simulink model "purepursuit"  (R2025a)
settings: Solver=VariableStepAuto  StartTime=0.0  StopTime=200  RelTol=1e-3
libraries: drivingscenarioandsensors x1, autolibshared x1
settings Model: Creator=bsb  LastModifiedBy=bsb

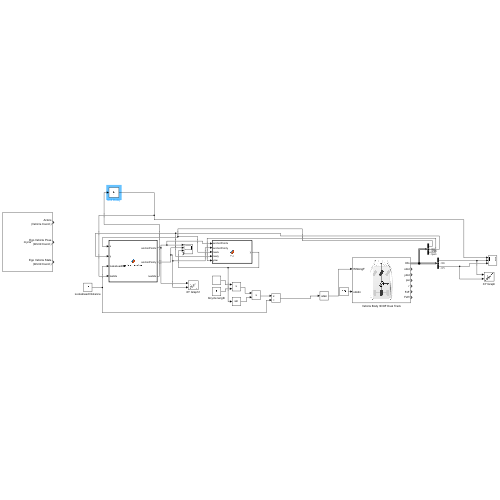
[thumbnail: Simulink's stored preview of the top-level diagram]
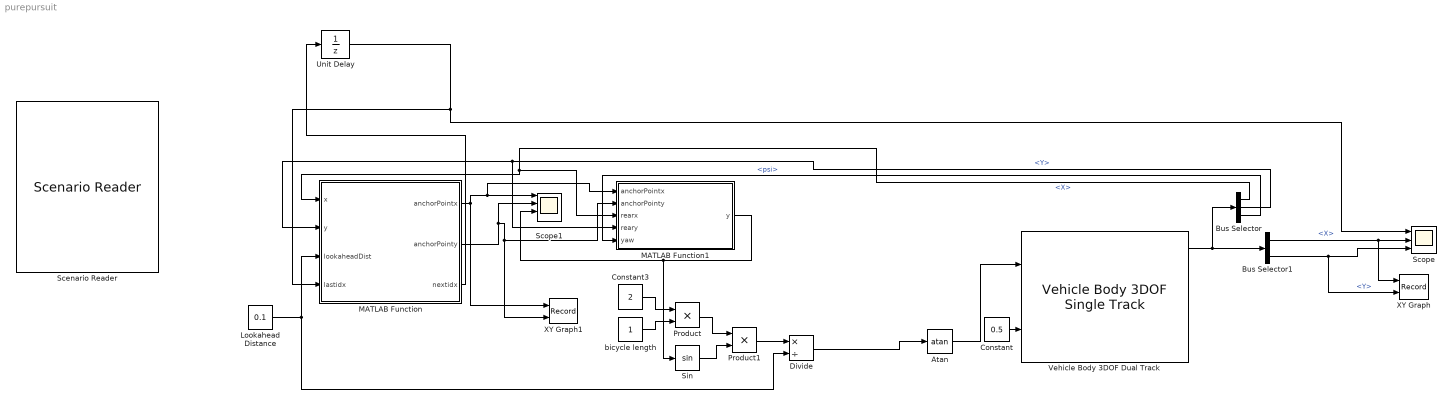
== system purepursuit ==
  Atan : Trigonometry  Operator=atan
  Bus Selector : BusSelector  OutputSignals=InertFrm.RearAxl.Disp.X,InertFrm.RearAxl.Disp.Y,InertFrm.Cg.Ang.psi
  Bus Selector1 : BusSelector  OutputSignals=InertFrm.Cg.Disp.X,InertFrm.Cg.Disp.Y
  Constant : Constant  Value=0.5
  Constant3 : Constant  Value=2
  Divide : Product  Inputs=*/
  Lookahead Distance : Constant  Value=0.1
  MATLAB Function : MATLAB Function  TreatAsAtomicUnit=on
  MATLAB Function1 : MATLAB Function  TreatAsAtomicUnit=on
  Product : Product
  Product1 : Product
  Scenario Reader : drivingscenarioandsensors/Scenario Reader  ScenarioSource=From file  ScenarioFileName=C:\Users\bsb\Documents\MATLAB\mycar.mat  ScenarioVariableName=scenario  OutputCoordinateSystem=Vehicle coordinates  EgoVehicleSource=Scenario  EgoVehicleActorID=1  OrientVehiclesOnRoad=off  OutputEgoVehiclePose=on  OutputEgoVehicleState=on  SampleTime=0.1  LaneBoundaryOutput=None  LaneBoundaryDistance=0:0.5:9.5  LaneBoundaryLocation=Center of lane markings  BusNameSource=Auto  BusName=BusActors  BusNumActorsSource=Scenario  BusNumActors=100  BusName2Source=Auto  BusName2=BusLaneBoundaries  BusNumLaneBoundariesSource=Scenario  BusNumLaneBoundaries=10  BusName3Source=Auto  BusName3=BusEgoActor  BusName4Source=Auto  BusName4=BusEgoState  ShowCoordinateLabels=on  SimulateUsing=Interpreted execution
  Scope : Scope  NumInputPorts=3
      settings: ActiveDisplayYMinimum=6.6611816133990995  ActiveDisplayYMaximum=22.945488903629986
  Scope1 : Scope  NumInputPorts=4
      settings: ActiveDisplayYMinimum=-0.018595181239648123  ActiveDisplayYMaximum=0.00095474296248539321
  Sin : Trigonometry
  Unit Delay : UnitDelay  SampleTime=-1  HasFrameUpgradeWarning=on
  Vehicle Body 3DOF Dual Track : autolibshared/Vehicle Body 3DOF Single Track  trackMode=Single (bicycle)  inputMode=External longitudinal velocity  frontSteerMode=on  rearSteerMode=off  windMode=off  muMode=off  extFMode=off  extMMode=off  htchFMode=off  htchMMode=off  extXo=off  extpsio=off  extxdoto=off  extro=off  extYo=off  extTamb=off  extydoto=off  aMode=2  NF=2  NR=2  m=2000  a=1.4  b=1.6  h=0.35  dh=1  hh=0.2  X_o=0  xdot_o=0  CalphaMode=off  sigmaMode=on  d=0  hl=0  w=[1.4,1.4]  Cy_f=12e3  Cy_r=11e3  sigma_f=.1  sigma_r=.1  alpha_f_brk=[-.1 .1]  Cy_f_data=[-9e3 9e3]  alpha_r_brk=[-.1 .1]  Cy_r_data=[-9e3 9e3]  Y_o=0  ydot_o=0  Izz=4000  psi_o=0  r_o=0  Af=2  Cd=.3  Cl=.1  Cpm=.1  beta_w=[0 0.01:0.01:0.3]  Cs=[0:0.03:0.9]  Cym=[0 1e-6:0.01:0.3]  Pabs=101325  Tair=273  g=9.81  mu=1  xdot_tol=.01  Fznom=5000  Fxtire_sat=7e4  Fytire_sat=7e4  longOff=0  latOff=0  vertOff=0  wrapAng=off
      settings: LibrarySourceBlock=vehdynlibeom/Vehicle Body 3DOF Dual Track
  XY Graph : Record  NumPorts=2.0  FileSettingsInternal="{\"entries\":[{\"content\":{\"excelSettings\":{\"content\":{},\"type\":\"Streamout.ExcelSettings\"},\"parquetSettings\":{\"content\":{},\"type\":\"Streamout.ParquetSettings\"}},\"type\":\"Streamout.FileSettingStorage\",\"uuid\":\"\"}],\"packageUris\":[\"http:\\/\\/schema.mathworks.com\\/mf0\\/streamout_blocks\\/R2020a\"],\"version\":\"1.0\"}"  FrameSettings=[0, 0]  Layout=[1 1]  SignalsInternal="{\"entries\":[{\"content\":{\"signals\":[{\"content\":{\"blockPath\":[],\"dimensions\":[1],\"domain\":\"\",\"lineColor\":\"#a2142f\",\"plots\":[ 1 ],\"port\":1,\"sid\":[\"\"],\"signalID\":1,\"signalName\":\"<X>\"},\"type\":\"RecordBlkView.Signal\",\"uuid\":\"\"},{\"content\":{\"blockPath\":[],\"dimensions\":[1],\"domain\":\"\",\"lineColor\":\"#139fff\",\"plots\":[ 1 ],\"port\":2,\"sid\":[\"\"],\"signalID\":2,\"signalName\":\"<Y>\"},\"type\":\"RecordBlkView.Signal\",\"uuid\":\"\"}]},\"type\":\"RecordBlkView.InputSignals\",\"uuid\":\"\"}],\"packageUris\":[\"http:\\/\\/schema.mathworks.com\\/mf0\\/streamout_blocks\\/R2020a\"],\"version\":\"1.0\"}"  VisualizationBindings="{\"xyplotplugin\":{\"info\":[{\"series\":[{\"bindingParametersList\":[{\"parameter\":\"X-Axis\",\"signalID\":1,\"signalName\":\"<X>\"},{\"parameter\":\"Y-Axis\",\"signalID\":2,\"signalName\":\"<Y>\"}],\"seriesID\":0}],\"subplotID\":1}]}}"  CompatibilityTag=XY
  XY Graph1 : Record  NumPorts=2.0  FileSettingsInternal="{\"entries\":[{\"content\":{\"excelSettings\":{\"content\":{},\"type\":\"Streamout.ExcelSettings\"},\"parquetSettings\":{\"content\":{},\"type\":\"Streamout.ParquetSettings\"}},\"type\":\"Streamout.FileSettingStorage\",\"uuid\":\"\"}],\"packageUris\":[\"http:\\/\\/schema.mathworks.com\\/mf0\\/streamout_blocks\\/R2020a\"],\"version\":\"1.0\"}"  FrameSettings=[0, 0]  Layout=[1 1]  SignalsInternal="{\"entries\":[{\"content\":{\"signals\":[{\"content\":{\"blockPath\":[],\"dimensions\":[1],\"domain\":\"\",\"lineColor\":\"#a2142f\",\"plots\":[ 1 ],\"port\":1,\"sid\":[\"\"],\"signalID\":1,\"signalName\":\"MATLAB Function:1\"},\"type\":\"RecordBlkView.Signal\",\"uuid\":\"\"},{\"content\":{\"blockPath\":[],\"dimensions\":[1],\"domain\":\"\",\"lineColor\":\"#139fff\",\"plots\":[ 1 ],\"port\":2,\"sid\":[\"\"],\"signalID\":2,\"signalName\":\"MATLAB Function:2\"},\"type\":\"RecordBlkView.Signal\",\"uuid\":\"\"}]},\"type\":\"RecordBlkView.InputSignals\",\"uuid\":\"\"}],\"packageUris\":[\"http:\\/\\/schema.mathworks.com\\/mf0\\/streamout_blocks\\/R2020a\"],\"version\":\"1.0\"}"  VisualizationBindings="{\"xyplotplugin\":{\"info\":[{\"series\":[{\"bindingParametersList\":[{\"parameter\":\"X-Axis\",\"signalID\":1,\"signalName\":\"MATLAB Function:1\"},{\"parameter\":\"Y-Axis\",\"signalID\":2,\"signalName\":\"MATLAB Function:2\"}],\"seriesID\":0}],\"subplotID\":1}]}}"  CompatibilityTag=XY
  bicycle length : Constant
  wires:
  Lookahead Distance/1 -> MATLAB Function/3(lookaheadDist), Divide/2
  Vehicle Body 3DOF Dual Track/1 -> Bus Selector1/1, Bus Selector/1
  bicycle length/1 -> Product/2
  Constant3/1 -> Product/1
  Product/1 -> Product1/1
  Sin/1 -> Product1/2
  Product1/1 -> Divide/1
  Divide/1 -> Atan/1
  Atan/1 -> Vehicle Body 3DOF Dual Track/1
  Bus Selector/1 -> MATLAB Function/1(x), MATLAB Function1/3(rearx)  "<X>"
  Constant/1 -> Vehicle Body 3DOF Dual Track/2
  MATLAB Function/1(anchorPointx) -> Scope1/1, MATLAB Function1/1(anchorPointx), XY Graph1/1
  MATLAB Function/2(anchorPointy) -> XY Graph1/2, MATLAB Function1/2(anchorPointy), Scope1/2
  Bus Selector/3 -> MATLAB Function1/5(yaw)  "<psi>"
  MATLAB Function1/1(y) -> Scope1/3, Sin/1
  Bus Selector1/2 -> XY Graph/2, Scope/3  "<Y>"
  Bus Selector1/1 -> XY Graph/1, Scope/2  "<X>"
  MATLAB Function/3(nextidx) -> Unit Delay/1
  Unit Delay/1 -> Scope/1, MATLAB Function/4(lastidx)
  Bus Selector/2 -> MATLAB Function/2(y), MATLAB Function1/4(reary)  "<Y>"

== matlab function purepursuit/MATLAB Function1 ==
  data: anchorPointx input; y output; anchorPointy input; rearx input; reary input; yaw input
function y = fcn(anchorPointx, anchorPointy, rearx, reary, yaw)
    v_car = [cos(yaw), sin(yaw)];
    anchor = [anchorPointx, anchorPointy];
    rearc = [rearx, reary];
    v_target = anchor - rearc;
    v_target = v_target / (norm(v_target) + 1e-6);
    crossval = v_car(1)*v_target(2) - v_car(2)*v_target(1);
    dotval = v_car(1)*v_target(1) + v_car(2)*v_target(2);
    y = atan2(crossval, dotval);
end

== matlab function purepursuit/MATLAB Function ==
  data: x input; anchorPointx output; y input; lookaheadDist input; lastidx input; anchorPointy output; nextidx output
function [anchorPointx, anchorPointy, nextidx] = getNextAnchor(x, y, lookaheadDist, lastidx)
%#codegen
% GETNEXTANCHOR  根据车辆位置和前视距离选取下一个锚点（基于累积弧长）
%   输入：
%     x, y           — 车辆当前位置（标量）
%     lookaheadDist — 前视距离（标量）
%     lastidx       — 上次选中的 waypoint 索引（标量）
%   输出：
%     anchorPointx  — 选中 waypoint 的 x 坐标（1×1 标量）
%     anchorPointy  — 选中 waypoint 的 y 坐标（1×1 标量）
%     nextidx       — 选中 waypoint 在列表中的行索引（1×1 标量）

    arguments (Input)
        x             (1,1) double
        y             (1,1) double
        lookaheadDist (1,1) double
        lastidx       (1,1) double
    end
    arguments (Output)
        anchorPointx  (1,1) double
        anchorPointy  (1,1) double
        nextidx       (1,1) double
    end

    waypoints = [ 
        0.8, -1.8;
        2.1, -4.2;
        4.1, -7.5;
        5.9,-11.6;
        8.2,-15.0;
       11.4,-18.0;
       14.2,-18.6;
       17.2,-18.2;
       20.1,-17.2;
       22.5,-14.8;
       24.6,-11.9;
       26.7, -8.9;
       28.4, -6.0;
       29.8, -3.0;
       31.2,  1.4;
       32.5,  5.4;
       34.3,  9.5;
       36.6, 12.0;
       39.3, 12.3;
       42.1, 10.1;
       44.6,  5.6;
       46.4,  1.5;
       47.6, -3.8;
       48.2, -9.9;
       49.1,-16.4 
    ];

    N = size(waypoints,1);
    if lastidx < 1 || lastidx > N
        lastidx = 1;
    end

    %—— 计算当前位置到路径上 lastidx 点的矢量，可选用于调试 ——%
    disp(hypot(waypoints(lastidx,1)-x, waypoints(lastidx,2)-y));

    %—— 沿路径累积弧长寻找下一个点 ——%
    cumDist = 0;  % 累加的路径长度
    nextidx = N;  % 默认选最后一个点
    for i = lastidx:(N-1)
        % 计算 waypoint i -> i+1 之间的段长
        dx = waypoints(i+1,1) - waypoints(i,1);
        dy = waypoints(i+1,2) - waypoints(i,2);
        segLen = hypot(dx, dy);
        cumDist = cumDist + segLen;
        if cumDist >= lookaheadDist
            nextidx = i + 1;
            break;
        end
    end

    %—— 如果当前点还是大于ld，还是选当前点而不是选择下一个点 ——%
    dx = waypoints(lastidx,1) - x;
    dy = waypoints(lastidx,2) - y;
    segLen = hypot(dx, dy);
    if segLen >= lookaheadDist
        nextidx = lastidx;
    end

    %—— 输出锚点坐标 ——%
    anchorPointx = waypoints(nextidx, 1);
    anchorPointy = waypoints(nextidx, 2);
end
